simulink model "chap9_7"  (Simulink 3.00)
settings: Solver=ode45  StartTime=0.0  StopTime=10  RelTol=1e-3
values from neighbouring files (symbols this model uses):
  b = 1    [Chap9_5i.m]    (also in chap9_7i.m = 0.5)
  f1 = (b+kd*kv)    (= 12.5)    [chap9_7i.m]
  f2 = J    (= 2)    [chap9_7i.m]
  J = 2    [Chap9_5i.m]    (also in chap9_1eq.m = 1; chap9_2i.m = 1; chap9_3.m = 0.6; chap9_4plant.m = 0.6)
  kd = 6    [Chap9_5i.m]    (also in chap9_6i.m; chap9_7i.m)
  kp = 15    [chap9_7i.m]
  kv = 2.0    (= 2)    [CHAP9_3F.M]    (also in Chap9_5i.m; chap9_4plant.m; chap9_6i.m; chap9_7i.m)

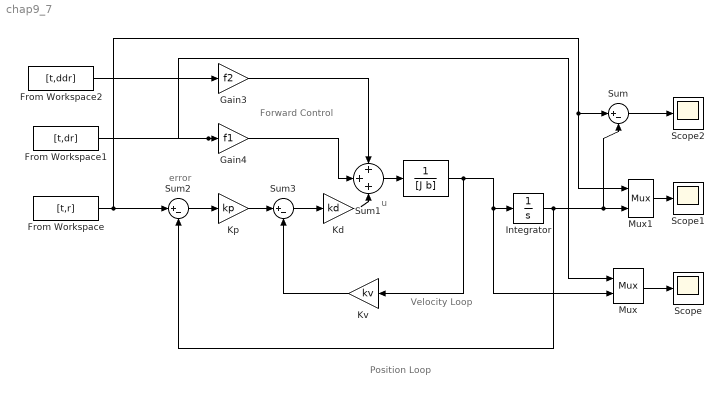
== system chap9_7 ==
  note: u
  note: Position Loop
  note: Velocity Loop
  note: Forward Control
  note: error
  " " : TransferFcn  Numerator=[1]  Denominator=[J b]
  From Workspace : FromWorkspace  VariableName=[t,r]  SampleTime=0.001  HoldFinalValue=off
  From Workspace1 : FromWorkspace  VariableName=[t,dr]  SampleTime=0.001  HoldFinalValue=off
  From Workspace2 : FromWorkspace  VariableName=[t,ddr]  SampleTime=0.001  HoldFinalValue=off
  Gain3 : Gain  Gain=f2  SaturateOnIntegerOverflow=off
  Gain4 : Gain  Gain=f1  SaturateOnIntegerOverflow=off
  Integrator : Integrator  ExternalReset=none  InitialConditionSource=internal  InitialCondition=0  LimitOutput=off  UpperSaturationLimit=inf  LowerSaturationLimit=-inf  ShowSaturationPort=off  ShowStatePort=off  AbsoluteTolerance=auto
  Kd : Gain  Gain=kd  SaturateOnIntegerOverflow=on
  Kp : Gain  Gain=kp  SaturateOnIntegerOverflow=on
  Kv : Gain  Orientation=left  Gain=kv  SaturateOnIntegerOverflow=on
  Mux : Mux  Inputs=2
      settings: DisplayOption=none
  Mux1 : Mux  Inputs=2
      settings: DisplayOption=none
  Scope : Scope
      settings: TimeRange=auto  YMin=-5  YMax=5  SaveToWorkspace=off  SaveName=ScopeData  MaxRows=50000
  Scope1 : Scope
      settings: TimeRange=auto  YMin=-1.1  YMax=1.1  SaveToWorkspace=off  SaveName=ScopeData  MaxRows=50000
  Scope2 : Scope
      settings: TimeRange=auto  YMin=-1.1  YMax=1.1  SaveToWorkspace=off  SaveName=ScopeData  MaxRows=50000
  Sum : Sum  Inputs=|+-  SaturateOnIntegerOverflow=on
  Sum1 : Sum  Inputs=+++  SaturateOnIntegerOverflow=off
  Sum2 : Sum  Inputs=|+-  SaturateOnIntegerOverflow=on
  Sum3 : Sum  Inputs=|+-  SaturateOnIntegerOverflow=on
  wires:
  Gain3/1 -> Sum1/1
  Sum2/1 -> Kp/1
  Kd/1 -> Sum1/3
  Kv/1 -> Sum3/2
  Sum3/1 -> Kd/1
  Kp/1 -> Sum3/1
  Gain4/1 -> Sum1/2
  Sum1/1 -> " "/1
  Mux/1 -> Scope/1
  Mux1/1 -> Scope1/1
  Integrator/1 -> Sum2/2, Mux1/2, Sum/2
  Sum/1 -> Scope2/1
  From Workspace2/1 -> Gain3/1
  From Workspace1/1 -> Gain4/1, Mux/1
  From Workspace/1 -> Sum2/1, Mux1/1, Sum/1
  " "/1 -> Integrator/1, Mux/2, Kv/1
